simulink model "testsim"  (R2018b)
settings: Solver=ode4  StartTime=0.0  StopTime=5  FixedStep=0.001  RelTol=1e-3  EnableMultiTasking=on
settings Model: ExtModeTrigMode=oneshot  ExtModeArmWhenConnect=off  Creator=hp  LastModifiedBy=Administrator
settings DataIOCC: SaveFormat=Array  SignalLoggingSaveFormat=ModelDataLogs  SignalLoggingName=sigsOut
settings OptimizationCC: BooleanDataType=off  ExpressionDepthLimit=2147483647  InitFltsAndDblsToZero=on  LifeSpan=inf
settings DebuggingCC: SaveWithParameterizedLinksMsg=none  UnderspecifiedInitializationDetection=Classic  MergeDetectMultiDrivingBlocksExec=none  SignalResolutionControl=TryResolveAllWithWarning  MultiTaskDSMMsg=warning  MultiTaskCondExecSysMsg=none  FcnCallInpInsideContextMsg=warning  StateNameClashWarn=warning  SFUnexpectedBacktrackingDiag=warning  SFNoUnconditionalDefaultTransitionDiag=warning  SFExecutionAtInitializationDiag=none
settings HardwareCC: ProdBitPerPointer=32  ProdBitPerSizeT=32  ProdBitPerPtrDiffT=32  ProdLargestAtomicFloat=None  ProdIntDivRoundTo=Undefined  ProdEndianess=Unspecified  ProdWordSize=32  ProdHWDeviceType=32-bit Generic  TargetUnknown=on
settings ModelReferenceCC: PropagateSignalLabelsOutOfModel=off
settings SFSimCC: SimUseLocalCustomCode=off
settings RTWCC: RTWUseLocalCustomCode=off
settings CodeAppCC: StateflowObjectComments=on
settings GRTTargetCC: TargetFcnLib=ansi_tfl_tmw.mat  TargetLangStandard=C89/C90 (ANSI)  GeneratePreprocessorConditionals=Disable all  CombineOutputUpdateFcns=off  GRTInterface=on
settings ConfigComp: CovMetricSettings=dw  CovHtmlReporting=on  CovSaveCumulativeToWorkspaceVar=on  CovSaveSingleToWorkspaceVar=on  CovExternalEMLEnable=off

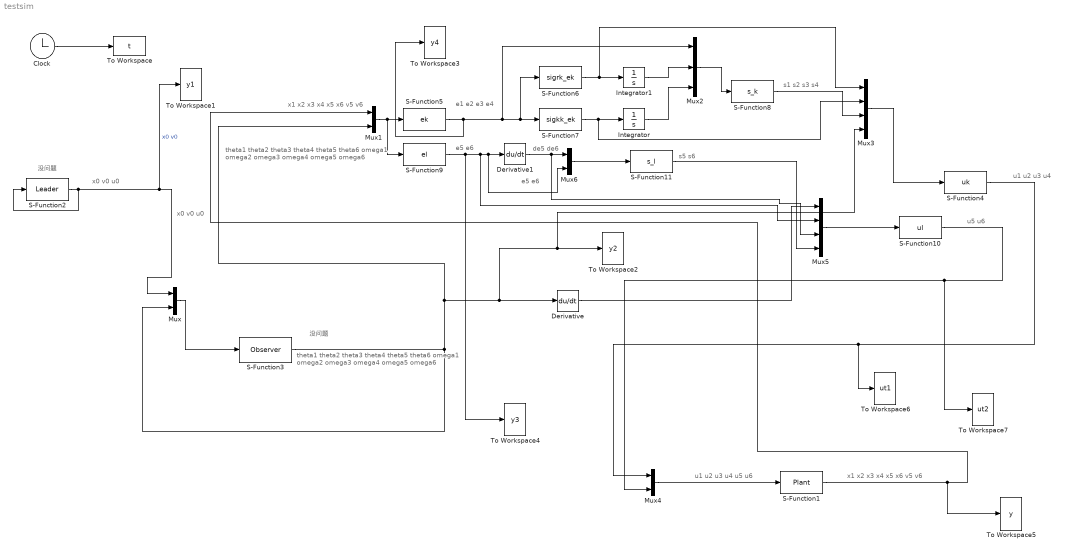
== system testsim ==
  note: s5 s6
  note: s1 s2 s3 s4
  note: de5 de6
  note: e1 e2 e3 e4
  note: e5 e6
  note: u1 u2 u3 u4 u5 u6
  note: u1 u2 u3 u4
  note: x1 x2 x3 x4 x5 x6 v5 v6
  note: x0 v0 u0
  note: 没问题
  note: 没问题
  note: x0 v0 u0
  note: theta1 theta2 theta3 theta4 theta5 theta6
      | omega1 omega2 omega3 omega4 omega5 omega6
  note: u5 u6
  note: theta1 theta2 theta3 theta4 theta5 theta6
      | omega1 omega2 omega3 omega4 omega5 omega6
  note: x1 x2 x3 x4 x5 x6 v5 v6
  note: e5 e6
  Clock : Clock
  Derivative : Derivative
  Derivative1 : Derivative
  Integrator : Integrator
  Integrator1 : Integrator
  Mux{,1,4,6} (4 alike) : Mux  Inputs=2
  Mux2 : Mux  Inputs=3
  Mux3 : Mux
  Mux5 : Mux
  S-Function1 : S-Function  FunctionName=Plant  SFunctionDeploymentMode=off  EnableBusSupport=off
  S-Function10 : S-Function  FunctionName=ul  SFunctionDeploymentMode=off  EnableBusSupport=off
  S-Function11 : S-Function  FunctionName=s_l  SFunctionDeploymentMode=off  EnableBusSupport=off
  S-Function2 : S-Function  FunctionName=Leader  SFunctionDeploymentMode=off  EnableBusSupport=off
  S-Function3 : S-Function  FunctionName=Observer  SFunctionDeploymentMode=off  EnableBusSupport=off
  S-Function4 : S-Function  FunctionName=uk  SFunctionDeploymentMode=off  EnableBusSupport=off
  S-Function5 : S-Function  FunctionName=ek  SFunctionDeploymentMode=off  EnableBusSupport=off
  S-Function6 : S-Function  FunctionName=sigrk_ek  SFunctionDeploymentMode=off  EnableBusSupport=off
  S-Function7 : S-Function  FunctionName=sigkk_ek  SFunctionDeploymentMode=off  EnableBusSupport=off
  S-Function8 : S-Function  FunctionName=s_k  SFunctionDeploymentMode=off  EnableBusSupport=off
  S-Function9 : S-Function  FunctionName=el  SFunctionDeploymentMode=off  EnableBusSupport=off
  To Workspace : ToWorkspace  VariableName=t  SampleTime=-1
  To Workspace1 : ToWorkspace  VariableName=y1  SampleTime=-1
  To Workspace2 : ToWorkspace  VariableName=y2  SampleTime=-1
  To Workspace3 : ToWorkspace  VariableName=y4  SampleTime=-1
  To Workspace4 : ToWorkspace  VariableName=y3  SampleTime=-1
  To Workspace5 : ToWorkspace  VariableName=y  SampleTime=-1
  To Workspace6 : ToWorkspace  VariableName=ut1  SampleTime=-1
  To Workspace7 : ToWorkspace  VariableName=ut2  SampleTime=-1
  wires:
  Clock/1 -> To Workspace/1
  S-Function2/1 -> Mux/1, To Workspace1/1, S-Function2/1  "x0 v0"
  Mux/1 -> S-Function3/1
  S-Function3/1 -> Mux3/4, To Workspace2/1, Derivative/1, Mux1/2, Mux/2
  Mux1/1 -> S-Function9/1, S-Function5/1
  S-Function1/1 -> To Workspace5/1, Mux1/1
  S-Function5/1 -> To Workspace3/1, Mux2/1, S-Function7/1, S-Function6/1
  S-Function7/1 -> Mux3/2, Integrator/1
  S-Function6/1 -> Mux3/1, Integrator1/1
  Mux2/1 -> S-Function8/1
  Integrator1/1 -> Mux2/2
  S-Function8/1 -> Mux3/3
  Mux3/1 -> S-Function4/1
  Mux4/1 -> S-Function1/1
  S-Function4/1 -> To Workspace6/1, Mux4/1
  S-Function10/1 -> To Workspace7/1, Mux4/2
  S-Function9/1 -> To Workspace4/1, Mux5/2, Mux6/2, Derivative1/1
  Derivative1/1 -> Mux6/1, Mux5/3
  Mux6/1 -> S-Function11/1
  Derivative/1 -> Mux5/1
  S-Function11/1 -> Mux5/4
  Mux5/1 -> S-Function10/1
  Integrator/1 -> Mux2/3
